simulink model "ball_and_plate_za_nn_2"  (R2018b)
settings: Solver=ode45  StartTime=0.0  StopTime=t_sim  RelTol=1e-3  EnableMultiTasking=on
values from neighbouring files (symbols this model uses):
  A_x = 0.05    [parametri.mat]    (also in proba_nn_simulink.m = 0.1; simulate_NOE_NARX_performance.mat = 0.1; simuliraj_kruznicu.m = radijus; test_nn_.m = 0.1)
  a_x = 0.388    [parametri.mat]    (also in simulate_NOE_NARX_performance.mat)
  A_y = 0.05    [parametri.mat]    (also in proba_nn_simulink.m = 0.1; simulate_NOE_NARX_performance.mat = 0.1; simuliraj_kruznicu.m = radijus; test_nn_.m = 0.1)
  a_y = 0.473    [parametri.mat]    (also in simulate_NOE_NARX_performance.mat)
  Ak_x = 0.1    [parametri.mat]    (also in simulate_NOE_NARX_performance.mat; simuliraj_kvadrat.m = stranica)
  Ak_y = 0.1    [parametri.mat]    (also in simulate_NOE_NARX_performance.mat; simuliraj_kvadrat.m = stranica)
  d = 2    [parametri.mat]    (also in simulate_NOE_NARX_performance.mat)
  Fc = 9.9675e-08    [parametri.mat]    (also in simulate_NOE_NARX_performance.mat)
  freq_x = 0.628318530718    [parametri.mat]    (also in simulate_NOE_NARX_performance.mat)
  freq_y = 0.628318530718    [parametri.mat]    (also in simulate_NOE_NARX_performance.mat)
  Fs = 1.9935e-07    [parametri.mat]    (also in simulate_NOE_NARX_performance.mat)
  g = 9.81    [parametri.mat]    (also in simulate_NOE_NARX_performance.mat)
  Jl = 7.48815837481e-05    [parametri.mat]    (also in simulate_NOE_NARX_performance.mat)
  konstanta = 0.1    [parametri.mat]    (also in simulate_NOE_NARX_performance.mat; simuliraj_kvadrat.m = 0.03)
  l = 0.1    [parametri.mat]    (also in simulate_NOE_NARX_performance.mat)
  ml = 0.0786597330257    [parametri.mat]    (also in simulate_NOE_NARX_performance.mat)
  odabir = 3    [proba_nn_simulink.m]    (also in simulate_NOE_NARX_performance.mat; simuliraj_kruznicu.m; simuliraj_kvadrat.m = 2; simuliraj_referenca.m = 1)
  period_x = 16    [parametri.mat]    (also in simulate_NOE_NARX_performance.mat)
  period_y = 16    [parametri.mat]    (also in simulate_NOE_NARX_performance.mat)
  phase_x = 1.57079632679    [parametri.mat]    (also in simulate_NOE_NARX_performance.mat)
  phase_y = 0    [parametri.mat]    (also in simulate_NOE_NARX_performance.mat)
  phasedelay_x = 0    [parametri.mat]    (also in simulate_NOE_NARX_performance.mat)
  phasedelay_y = 4    [parametri.mat]    (also in simulate_NOE_NARX_performance.mat)
  pw_x = 50    [parametri.mat]    (also in simulate_NOE_NARX_performance.mat)
  pw_y = 50    [parametri.mat]    (also in simulate_NOE_NARX_performance.mat)
  R = 0.0397    [parametri.mat]    (also in simulate_NOE_NARX_performance.mat)
  r = 0.02    [parametri.mat]    (also in simulate_NOE_NARX_performance.mat)
  t_step = 5    [parametri.mat]    (also in simulate_NOE_NARX_performance.mat)
  Td = 0.1    [parametri.mat]    (also in simulate_NOE_NARX_performance.mat)
  vs = 0.05    [parametri.mat]    (also in simulate_NOE_NARX_performance.mat)
  x0 = 0.15    [parametri.mat]    (also in proba_nn_simulink.m = a_x/2.0; simulate_NOE_NARX_performance.mat = 0.194; simuliraj_kruznicu.m = a_x/2.0; test_nn_.m = a_x/2.0)
  x0_loptica = 0.1    [proba_nn_simulink.m]    (also in simulate_NOE_NARX_performance.mat; simuliraj_kruznicu.m = x0_poc; simuliraj_kvadrat.m = x0_poc; simuliraj_referenca.m = x0_poc)
  x_step = 0.05    [parametri.mat]    (also in simulate_NOE_NARX_performance.mat; simuliraj_referenca.m = x_ref_value)
  y0 = 0.15    [parametri.mat]    (also in proba_nn_simulink.m = a_y/2.0; simulate_NOE_NARX_performance.mat = 0.2365; simuliraj_kruznicu.m = a_y/2.0; test_nn_.m = a_y/2.0)
  y0_loptica = 0.1    [proba_nn_simulink.m]    (also in simulate_NOE_NARX_performance.mat; simuliraj_kruznicu.m = y0_poc; simuliraj_kvadrat.m = y0_poc; simuliraj_referenca.m = y0_poc)
  y_step = 0.05    [parametri.mat]    (also in simulate_NOE_NARX_performance.mat; simuliraj_referenca.m = y_ref_value)
libraries: neural x118, simulink x6, fuzblock x2
(part 1 of 5)
settings Model: SimulationMode=accelerator  Creator=Damjan  LastModifiedBy=branko
settings DataIOCC: LimitDataPoints=on  SaveFormat=Array  SignalLoggingSaveFormat=ModelDataLogs
settings OptimizationCC: ExpressionDepthLimit=2147483647  LifeSpan=inf
settings DebuggingCC: UnderspecifiedInitializationDetection=Classic  MergeDetectMultiDrivingBlocksExec=none  FcnCallInpInsideContextMsg=warning  AllowSymbolicDim=off  StateNameClashWarn=warning  SFUnexpectedBacktrackingDiag=warning  SFNoUnconditionalDefaultTransitionDiag=warning  SFExecutionAtInitializationDiag=none
settings HardwareCC: ProdBitPerPointer=32  ProdBitPerSizeT=32  ProdBitPerPtrDiffT=32  ProdLargestAtomicFloat=None  ProdIntDivRoundTo=Undefined  ProdEndianess=Unspecified  ProdWordSize=32  ProdHWDeviceType=32-bit Generic
settings ModelReferenceCC: PropagateSignalLabelsOutOfModel=off
settings SFSimCC: SimUseLocalCustomCode=off
settings RTWCC: RTWUseLocalCustomCode=off
settings CodeAppCC: StateflowObjectComments=on
settings GRTTargetCC: TargetLangStandard=C89/C90 (ANSI)  GeneratePreprocessorConditionals=Disable all  CombineOutputUpdateFcns=off  GRTInterface=on
settings ConfigComp: CovMetricSettings=dw  CovHtmlReporting=on  CovSaveCumulativeToWorkspaceVar=on  CovSaveSingleToWorkspaceVar=on  CovExternalEMLEnable=off

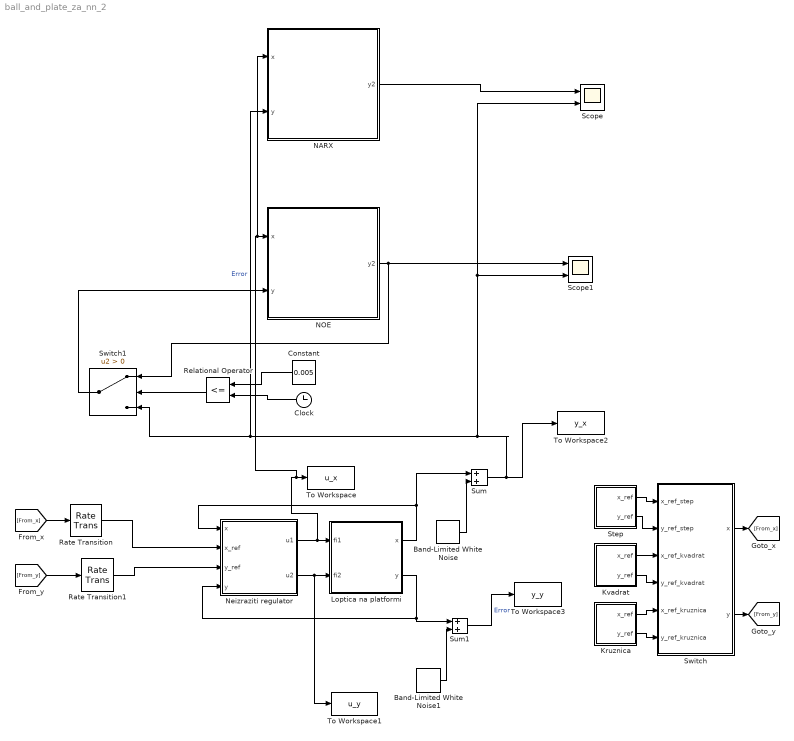
== system ball_and_plate_za_nn_2 ==
  Band-Limited White Noise : simulink/Sources/Band-Limited White Noise  Cov=[1e-9]  Ts=0.001  seed=[23341]
  Band-Limited White Noise1 : simulink/Sources/Band-Limited White Noise  Cov=[1e-9]  Ts=0.001  seed=[23341]
  Clock : Clock
  Constant : Constant  Value=0.005  OutDataTypeStr=double  SampleTime=-1
  Kruznica : Subsystem
  Kvadrat : Subsystem
  Loptica na platformi : Subsystem
  NARX : Subsystem  mask{pi_input_1_delayed_1=0, pi_input_1_delayed_2=0, pi_input_1_delayed_3=0, pi_input_1_delayed_4=0, pi_input_1_delayed_5=0, pi_input_2_delayed_1=0, pi_input_2_delayed_2=0, pi_input_2_delayed_3=0, pi_input_2_delayed_4=0, pi_input_2_delayed_5=0}
      mask prompts: pi_input_1_delayed_1 "Preprocessed initial input 1 state at timestep 0."; pi_input_1_delayed_2 "Preprocessed initial input 1 state at timestep -1."; pi_input_1_delayed_3 "Preprocessed initial input 1 state at timestep -2."; pi_input_1_delayed_4 "Preprocessed initial input 1 state at timestep -3."; pi_input_1_delayed_5 "Preprocessed initial input 1 state at timestep -4."; pi_input_2_delayed_1 "Preprocessed initial input 2 state at timestep 0."; pi_input_2_delayed_2 "Preprocessed initial input 2 state at timestep -1."; pi_input_2_delayed_3 "Preprocessed initial input 2 state at timestep -2."; pi_input_2_delayed_4 "Preprocessed initial input 2 state at timestep -3."; pi_input_2_delayed_5 "Preprocessed initial input 2 state at timestep -4."
      mask help: NARX Neural Network
      mask Display: e = 0.06;c1 = [120 150 230]/255;c2 = ([120 150 230]+0)/383;c3 = ([120 150 230]+128)/383;patch([0 1 1 0],[0 0 1 1],c1);patch([0 1 1 1-e 1-e 0+e],[0 0 1 1-e 0+e 0+e],c2);patch([0 0 1 1-e 0+e 0+e],[0 1 1 1-e 1-e 0+e],c3);plot([0 1 1 0 0],[0 0 1 1 0]);fprintf('NNET');port_label('input',1,' x');port_label('input',2,' y');port_label('output',1,'y2 ');
  NOE : Subsystem  mask{pi_input_1_delayed_1=0, pi_input_1_delayed_2=0, pi_input_1_delayed_3=0, pi_input_1_delayed_4=0, pi_input_1_delayed_5=0, pi_input_2_delayed_1=0, pi_input_2_delayed_2=0, pi_input_2_delayed_3=0, pi_input_2_delayed_4=0, pi_input_2_delayed_5=0}
      mask prompts: pi_input_1_delayed_1 "Preprocessed initial input 1 state at timestep 0."; pi_input_1_delayed_2 "Preprocessed initial input 1 state at timestep -1."; pi_input_1_delayed_3 "Preprocessed initial input 1 state at timestep -2."; pi_input_1_delayed_4 "Preprocessed initial input 1 state at timestep -3."; pi_input_1_delayed_5 "Preprocessed initial input 1 state at timestep -4."; pi_input_2_delayed_1 "Preprocessed initial input 2 state at timestep 0."; pi_input_2_delayed_2 "Preprocessed initial input 2 state at timestep -1."; pi_input_2_delayed_3 "Preprocessed initial input 2 state at timestep -2."; pi_input_2_delayed_4 "Preprocessed initial input 2 state at timestep -3."; pi_input_2_delayed_5 "Preprocessed initial input 2 state at timestep -4."
      mask help: NARX Neural Network
      mask Display: e = 0.06;c1 = [120 150 230]/255;c2 = ([120 150 230]+0)/383;c3 = ([120 150 230]+128)/383;patch([0 1 1 0],[0 0 1 1],c1);patch([0 1 1 1-e 1-e 0+e],[0 0 1 1-e 0+e 0+e],c2);patch([0 0 1 1-e 0+e 0+e],[0 1 1 1-e 1-e 0+e],c3);plot([0 1 1 0 0],[0 0 1 1 0]);fprintf('NNET');port_label('input',1,' x');port_label('input',2,' y');port_label('output',1,'y2 ');
  Neizraziti regulator : Subsystem
  Rate Transition : RateTransition  OutPortSampleTime=0.001
  Rate Transition1 : RateTransition  OutPortSampleTime=0.001
  Relational Operator : RelationalOperator  Operator=<=  OutDataTypeStr=boolean  RndMeth=Simplest
  Scope : Scope  NumInputPorts=2
  Scope1 : Scope  NumInputPorts=2
  Step : Subsystem
  Sum : Sum
  Sum1 : Sum
  Switch : Subsystem
  Switch1 : Switch  Criteria=u2 > Threshold
  To Workspace : ToWorkspace  VariableName=u_x  SaveFormat=Structure With Time  SampleTime=0.001
  To Workspace1 : ToWorkspace  VariableName=u_y  SaveFormat=Structure With Time  SampleTime=0.001
  To Workspace2 : ToWorkspace  VariableName=y_x  SaveFormat=Structure With Time  SampleTime=0.001
  To Workspace3 : ToWorkspace  VariableName=y_y  SaveFormat=Structure With Time  SampleTime=0.001
  wires:
  Loptica na platformi/1(x) -> Sum/1, Neizraziti regulator/1(x)
  Loptica na platformi/2(y) -> Sum1/1, Neizraziti regulator/4(y)
  Neizraziti regulator/1(u1) -> NARX/1(x), NOE/1(x), To Workspace/1, Loptica na platformi/1(fi1)
  Neizraziti regulator/2(u2) -> To Workspace1/1, Loptica na platformi/2(fi2)
  [From_x] -> Rate Transition/1
  [From_y] -> Rate Transition1/1
  Switch/1(x) -> [From_x]
  Switch/2(y) -> [From_y]
  Step/1(x_ref) -> Switch/1(x_ref_step)
  Step/2(y_ref) -> Switch/2(y_ref_step)
  Kvadrat/1(x_ref) -> Switch/3(x_ref_kvadrat)
  Kvadrat/2(y_ref) -> Switch/4(y_ref_kvadrat)
  Kruznica/1(x_ref) -> Switch/5(x_ref_kruznica)
  Kruznica/2(y_ref) -> Switch/6(y_ref_kruznica)
  Band-Limited White Noise/1 -> Sum/2
  Sum/1 -> Scope1/2, Scope/2, NARX/2(y), Switch1/3, To Workspace2/1  "Error"
  Band-Limited White Noise1/1 -> Sum1/2
  Sum1/1 -> To Workspace3/1  "Error"
  Constant/1 -> Relational Operator/1
  Clock/1 -> Relational Operator/2
  Relational Operator/1 -> Switch1/2
  NOE/1(y2) -> Scope1/1, Switch1/1
  Switch1/1 -> NOE/2(y)
  Rate Transition/1 -> Neizraziti regulator/2(x_ref)
  Rate Transition1/1 -> Neizraziti regulator/3(y_ref)
  NARX/1(y2) -> Scope/1

== system ball_and_plate_za_nn_2/Kruznica ==
  Sinus x : Sin  Amplitude=A_x  Bias=x0  Frequency=freq_x  Phase=phase_x  SampleTime=0
  Sinus y : Sin  Amplitude=A_y  Bias=y0  Frequency=freq_y  Phase=phase_y  SampleTime=0
  x_ref : Outport
  y_ref : Outport  Port=2
  wires:
  Sinus x/1 -> x_ref/1
  Sinus y/1 -> y_ref/1

== system ball_and_plate_za_nn_2/Kvadrat ==
  Pulse Generator_x : DiscretePulseGenerator  PulseType=Time based  Amplitude=Ak_x  Period=period_x  PulseWidth=pw_x  PhaseDelay=phasedelay_x
  Pulse Generator_y : DiscretePulseGenerator  PulseType=Time based  Amplitude=Ak_y  Period=period_y  PulseWidth=pw_y  PhaseDelay=phasedelay_y
  Sum : Sum  Inputs=|++
  Sum1 : Sum  Inputs=|++
  const : Constant  Value=konstanta
  x_ref : Outport
  y_ref : Outport  Port=2
  wires:
  Sum/1 -> x_ref/1
  Sum1/1 -> y_ref/1
  Pulse Generator_x/1 -> Sum/1
  Pulse Generator_y/1 -> Sum1/1
  const/1 -> Sum1/2, Sum/2

== system ball_and_plate_za_nn_2/Loptica na platformi ==
  fi1 : Inport
  fi2 : Inport  Port=2
  Loptica : Subsystem
  Platforma : Subsystem
  x : Outport
  y : Outport  Port=2
  wires:
  Loptica/1(x) -> x/1
  fi1/1 -> Platforma/1(fi1)
  fi2/1 -> Platforma/2(fi2)
  Loptica/2(y) -> y/1
  Platforma/2(alfa) -> Loptica/2(alfa)
  Platforma/1(beta) -> Loptica/1(beta)

== system ball_and_plate_za_nn_2/NARX ==
  x : Inport  PortDimensions=1  SampleTime=0.001
      mask Display: e = 0.06;c1 = [120 230 180]/255;c2 = ([120 230 180]+0)/(256+128);c3 = ([120 230 180]+128)/(256+128);patch([0 1 1 0],[0 0 1 1],c1);patch([0 1 1 1-e 1-e 0+e],[0 0 1 1-e 0+e 0+e],c2);patch([0 0 1 1-e 0+e 0+e],[0 1 1 1-e 1-e 0+e],c3);plot([0 1 1 0 0],[0 0 1 1 0]);
  y : Inport  Port=2  PortDimensions=1  SampleTime=0.001
      mask Display: e = 0.06;c1 = [120 230 180]/255;c2 = ([120 230 180]+0)/(256+128);c3 = ([120 230 180]+128)/(256+128);patch([0 1 1 0],[0 0 1 1],c1);patch([0 1 1 1-e 1-e 0+e],[0 0 1 1-e 0+e 0+e],c2);patch([0 0 1 1-e 0+e 0+e],[0 1 1 1-e 1-e 0+e],c3);plot([0 1 1 0 0],[0 0 1 1 0]);
  Layer 1 : Subsystem
      mask Display: e = 0.06;c1 = [120 150 230]/255;c2 = ([120 150 230]+0)/383;c3 = ([120 150 230]+128)/383;patch([0 1 1 0],[0 0 1 1],c1);patch([0 1 1 1-e 1-e 0+e],[0 0 1 1-e 0+e 0+e],c2);patch([0 0 1 1-e 0+e 0+e],[0 1 1 1-e 1-e 0+e],c3);plot([0 1 1 0 0],[0 0 1 1 0]);
  Layer 2 : Subsystem
      mask Display: e = 0.06;c1 = [120 150 230]/255;c2 = ([120 150 230]+0)/383;c3 = ([120 150 230]+128)/383;patch([0 1 1 0],[0 0 1 1],c1);patch([0 1 1 1-e 1-e 0+e],[0 0 1 1-e 0+e 0+e],c2);patch([0 0 1 1-e 0+e 0+e],[0 1 1 1-e 1-e 0+e],c3);plot([0 1 1 0 0],[0 0 1 1 0]);
  Layer 3 : Subsystem
      mask Display: e = 0.06;c1 = [120 150 230]/255;c2 = ([120 150 230]+0)/383;c3 = ([120 150 230]+128)/383;patch([0 1 1 0],[0 0 1 1],c1);patch([0 1 1 1-e 1-e 0+e],[0 0 1 1-e 0+e 0+e],c2);patch([0 0 1 1-e 0+e 0+e],[0 1 1 1-e 1-e 0+e],c3);plot([0 1 1 0 0],[0 0 1 1 0]);
  Layer 4 : Subsystem
      mask Display: e = 0.06;c1 = [120 150 230]/255;c2 = ([120 150 230]+0)/383;c3 = ([120 150 230]+128)/383;patch([0 1 1 0],[0 0 1 1],c1);patch([0 1 1 1-e 1-e 0+e],[0 0 1 1-e 0+e 0+e],c2);patch([0 0 1 1-e 0+e 0+e],[0 1 1 1-e 1-e 0+e],c3);plot([0 1 1 0 0],[0 0 1 1 0]);
  Layer 5 : Subsystem
      mask Display: e = 0.06;c1 = [120 150 230]/255;c2 = ([120 150 230]+0)/383;c3 = ([120 150 230]+128)/383;patch([0 1 1 0],[0 0 1 1],c1);patch([0 1 1 1-e 1-e 0+e],[0 0 1 1-e 0+e 0+e],c2);patch([0 0 1 1-e 0+e 0+e],[0 1 1 1-e 1-e 0+e],c3);plot([0 1 1 0 0],[0 0 1 1 0]);
  Process Input 1 : Subsystem
      mask Display: e = 0.06;c1 = [120 150 230]/255;c2 = ([120 150 230]+0)/383;c3 = ([120 150 230]+128)/383;patch([0 1 1 0],[0 0 1 1],c1);patch([0 1 1 1-e 1-e 0+e],[0 0 1 1-e 0+e 0+e],c2);patch([0 0 1 1-e 0+e 0+e],[0 1 1 1-e 1-e 0+e],c3);plot([0 1 1 0 0],[0 0 1 1 0]);
  Process Input 2 : Subsystem
      mask Display: e = 0.06;c1 = [120 150 230]/255;c2 = ([120 150 230]+0)/383;c3 = ([120 150 230]+128)/383;patch([0 1 1 0],[0 0 1 1],c1);patch([0 1 1 1-e 1-e 0+e],[0 0 1 1-e 0+e 0+e],c2);patch([0 0 1 1-e 0+e 0+e],[0 1 1 1-e 1-e 0+e],c3);plot([0 1 1 0 0],[0 0 1 1 0]);
  Process Output 1 : Subsystem
      mask Display: e = 0.06;c1 = [120 150 230]/255;c2 = ([120 150 230]+0)/383;c3 = ([120 150 230]+128)/383;patch([0 1 1 0],[0 0 1 1],c1);patch([0 1 1 1-e 1-e 0+e],[0 0 1 1-e 0+e 0+e],c2);patch([0 0 1 1-e 0+e 0+e],[0 1 1 1-e 1-e 0+e],c3);plot([0 1 1 0 0],[0 0 1 1 0]);
  y2 : Outport  InitialOutput=0
      mask Display: e = 0.06;c1 = [120 230 180]/255;c2 = ([120 230 180]+0)/(256+128);c3 = ([120 230 180]+128)/(256+128);patch([0 1 1 0],[0 0 1 1],c1);patch([0 1 1 1-e 1-e 0+e],[0 0 1 1-e 0+e 0+e],c2);patch([0 0 1 1-e 0+e 0+e],[0 1 1 1-e 1-e 0+e],c3);plot([0 1 1 0 0],[0 0 1 1 0]);
  wires:
  x/1 -> Process Input 1/1(x)
  y/1 -> Process Input 2/1(x)
  Process Output 1/1(y) -> y2/1
  Process Input 1/1(p) -> Layer 1/1("p{1}")
  Process Input 2/1(p) -> Layer 1/2("p{2}")
  Layer 1/1("a{1}") -> [feedback1]
  [feedback1] -> Layer 2/1("a{1} ")
  Layer 2/1("a{2}") -> [feedback2]
  [feedback2] -> Layer 3/1("a{2} ")
  Layer 3/1("a{3}") -> [feedback3]
  [feedback3] -> Layer 4/1("a{3} ")
  Layer 4/1("a{4}") -> [feedback4]
  [feedback4] -> Layer 5/1("a{4} ")
  Layer 5/1("a{5}") -> Process Output 1/1(a)

== system ball_and_plate_za_nn_2/NOE ==
  x : Inport  PortDimensions=1  SampleTime=0.001
      mask Display: e = 0.06;c1 = [120 230 180]/255;c2 = ([120 230 180]+0)/(256+128);c3 = ([120 230 180]+128)/(256+128);patch([0 1 1 0],[0 0 1 1],c1);patch([0 1 1 1-e 1-e 0+e],[0 0 1 1-e 0+e 0+e],c2);patch([0 0 1 1-e 0+e 0+e],[0 1 1 1-e 1-e 0+e],c3);plot([0 1 1 0 0],[0 0 1 1 0]);
  y : Inport  Port=2  PortDimensions=1  SampleTime=0.001
      mask Display: e = 0.06;c1 = [120 230 180]/255;c2 = ([120 230 180]+0)/(256+128);c3 = ([120 230 180]+128)/(256+128);patch([0 1 1 0],[0 0 1 1],c1);patch([0 1 1 1-e 1-e 0+e],[0 0 1 1-e 0+e 0+e],c2);patch([0 0 1 1-e 0+e 0+e],[0 1 1 1-e 1-e 0+e],c3);plot([0 1 1 0 0],[0 0 1 1 0]);
  Layer 1 : Subsystem
      mask Display: e = 0.06;c1 = [120 150 230]/255;c2 = ([120 150 230]+0)/383;c3 = ([120 150 230]+128)/383;patch([0 1 1 0],[0 0 1 1],c1);patch([0 1 1 1-e 1-e 0+e],[0 0 1 1-e 0+e 0+e],c2);patch([0 0 1 1-e 0+e 0+e],[0 1 1 1-e 1-e 0+e],c3);plot([0 1 1 0 0],[0 0 1 1 0]);
  Layer 2 : Subsystem
      mask Display: e = 0.06;c1 = [120 150 230]/255;c2 = ([120 150 230]+0)/383;c3 = ([120 150 230]+128)/383;patch([0 1 1 0],[0 0 1 1],c1);patch([0 1 1 1-e 1-e 0+e],[0 0 1 1-e 0+e 0+e],c2);patch([0 0 1 1-e 0+e 0+e],[0 1 1 1-e 1-e 0+e],c3);plot([0 1 1 0 0],[0 0 1 1 0]);
  Layer 3 : Subsystem
      mask Display: e = 0.06;c1 = [120 150 230]/255;c2 = ([120 150 230]+0)/383;c3 = ([120 150 230]+128)/383;patch([0 1 1 0],[0 0 1 1],c1);patch([0 1 1 1-e 1-e 0+e],[0 0 1 1-e 0+e 0+e],c2);patch([0 0 1 1-e 0+e 0+e],[0 1 1 1-e 1-e 0+e],c3);plot([0 1 1 0 0],[0 0 1 1 0]);
  Layer 4 : Subsystem
      mask Display: e = 0.06;c1 = [120 150 230]/255;c2 = ([120 150 230]+0)/383;c3 = ([120 150 230]+128)/383;patch([0 1 1 0],[0 0 1 1],c1);patch([0 1 1 1-e 1-e 0+e],[0 0 1 1-e 0+e 0+e],c2);patch([0 0 1 1-e 0+e 0+e],[0 1 1 1-e 1-e 0+e],c3);plot([0 1 1 0 0],[0 0 1 1 0]);
  Layer 5 : Subsystem
      mask Display: e = 0.06;c1 = [120 150 230]/255;c2 = ([120 150 230]+0)/383;c3 = ([120 150 230]+128)/383;patch([0 1 1 0],[0 0 1 1],c1);patch([0 1 1 1-e 1-e 0+e],[0 0 1 1-e 0+e 0+e],c2);patch([0 0 1 1-e 0+e 0+e],[0 1 1 1-e 1-e 0+e],c3);plot([0 1 1 0 0],[0 0 1 1 0]);
  Process Input 1 : Subsystem
      mask Display: e = 0.06;c1 = [120 150 230]/255;c2 = ([120 150 230]+0)/383;c3 = ([120 150 230]+128)/383;patch([0 1 1 0],[0 0 1 1],c1);patch([0 1 1 1-e 1-e 0+e],[0 0 1 1-e 0+e 0+e],c2);patch([0 0 1 1-e 0+e 0+e],[0 1 1 1-e 1-e 0+e],c3);plot([0 1 1 0 0],[0 0 1 1 0]);
  Process Input 2 : Subsystem
      mask Display: e = 0.06;c1 = [120 150 230]/255;c2 = ([120 150 230]+0)/383;c3 = ([120 150 230]+128)/383;patch([0 1 1 0],[0 0 1 1],c1);patch([0 1 1 1-e 1-e 0+e],[0 0 1 1-e 0+e 0+e],c2);patch([0 0 1 1-e 0+e 0+e],[0 1 1 1-e 1-e 0+e],c3);plot([0 1 1 0 0],[0 0 1 1 0]);
  Process Output 1 : Subsystem
      mask Display: e = 0.06;c1 = [120 150 230]/255;c2 = ([120 150 230]+0)/383;c3 = ([120 150 230]+128)/383;patch([0 1 1 0],[0 0 1 1],c1);patch([0 1 1 1-e 1-e 0+e],[0 0 1 1-e 0+e 0+e],c2);patch([0 0 1 1-e 0+e 0+e],[0 1 1 1-e 1-e 0+e],c3);plot([0 1 1 0 0],[0 0 1 1 0]);
  y2 : Outport  InitialOutput=0
      mask Display: e = 0.06;c1 = [120 230 180]/255;c2 = ([120 230 180]+0)/(256+128);c3 = ([120 230 180]+128)/(256+128);patch([0 1 1 0],[0 0 1 1],c1);patch([0 1 1 1-e 1-e 0+e],[0 0 1 1-e 0+e 0+e],c2);patch([0 0 1 1-e 0+e 0+e],[0 1 1 1-e 1-e 0+e],c3);plot([0 1 1 0 0],[0 0 1 1 0]);
  wires:
  x/1 -> Process Input 1/1(x)
  y/1 -> Process Input 2/1(x)
  Process Output 1/1(y) -> y2/1
  Process Input 1/1(p) -> Layer 1/1("p{1}")
  Process Input 2/1(p) -> Layer 1/2("p{2}")
  Layer 1/1("a{1}") -> [feedback1]
  [feedback1] -> Layer 2/1("a{1} ")
  Layer 2/1("a{2}") -> [feedback2]
  [feedback2] -> Layer 3/1("a{2} ")
  Layer 3/1("a{3}") -> [feedback3]
  [feedback3] -> Layer 4/1("a{3} ")
  Layer 4/1("a{4}") -> [feedback4]
  [feedback4] -> Layer 5/1("a{4} ")
  Layer 5/1("a{5}") -> Process Output 1/1(a)

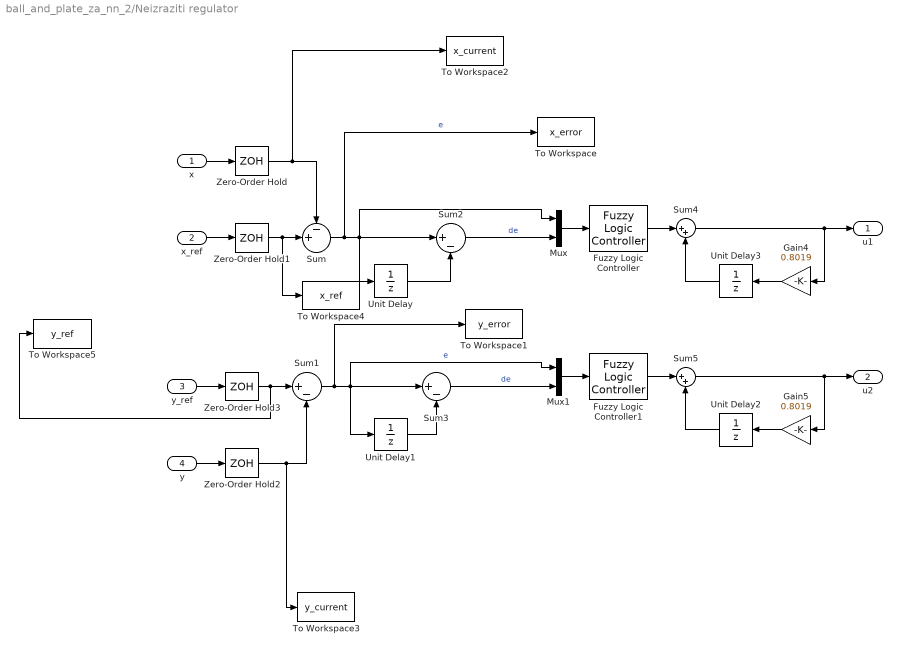
== system ball_and_plate_za_nn_2/Neizraziti regulator ==
  x : Inport
  x_ref : Inport  Port=2
  y_ref : Inport  Port=3
  y : Inport  Port=4
  Fuzzy Logic Controller : fuzblock/Fuzzy Logic  Controller  FIS=fuzzy_FIS  OutputSampleNumber=101  DataType=double  FuzzifiedInputs=off  RuleFiringStrengths=off  RuleOutputs=off  AggregatedOutputs=off  SimulateUsing=Interpreted execution  OutOfRangeInputValueMessage=warning  NoRuleFiredMessage=warning  EmptyOutputFuzzySetMessage=warning
  Fuzzy Logic Controller1 : fuzblock/Fuzzy Logic  Controller  FIS=fuzzy_FIS  OutputSampleNumber=101  DataType=double  FuzzifiedInputs=off  RuleFiringStrengths=off  RuleOutputs=off  AggregatedOutputs=off  SimulateUsing=Interpreted execution  OutOfRangeInputValueMessage=warning  NoRuleFiredMessage=warning  EmptyOutputFuzzySetMessage=warning
  Gain4 : Gain  Gain=0.8019
  Gain5 : Gain  Gain=0.8019
  Mux : Mux  Inputs=2
  Mux1 : Mux  Inputs=2
  Sum : Sum  Inputs=-+|  RndMeth=Nearest
  Sum1 : Sum  Inputs=|+-  RndMeth=Nearest
  Sum2 : Sum  Inputs=|+-
  Sum3 : Sum  Inputs=|+-
  Sum4 : Sum  Inputs=|++
  Sum5 : Sum  Inputs=|++
  To Workspace : ToWorkspace  VariableName=x_error  SaveFormat=Structure With Time  SampleTime=0.001
  To Workspace1 : ToWorkspace  VariableName=y_error  SaveFormat=Structure With Time  SampleTime=0.001
  To Workspace2 : ToWorkspace  VariableName=x_current  SaveFormat=Structure With Time  SampleTime=0.001
  To Workspace3 : ToWorkspace  VariableName=y_current  SaveFormat=Structure With Time  SampleTime=0.001
  To Workspace4 : ToWorkspace  VariableName=x_ref  SaveFormat=Structure With Time  SampleTime=0.001
  To Workspace5 : ToWorkspace  VariableName=y_ref  SaveFormat=Structure With Time  SampleTime=0.001
  Unit Delay : UnitDelay  SampleTime=-1
  Unit Delay1 : UnitDelay  SampleTime=-1
  Unit Delay2 : UnitDelay  SampleTime=Td
  Unit Delay3 : UnitDelay  SampleTime=Td
  Zero-Order Hold{,1..3} (4 alike) : ZeroOrderHold  SampleTime=Td
  u1 : Outport
  u2 : Outport  Port=2
  wires:
  x/1 -> Zero-Order Hold/1
  x_ref/1 -> Zero-Order Hold1/1
  y_ref/1 -> Zero-Order Hold3/1
  y/1 -> Zero-Order Hold2/1
  Zero-Order Hold/1 -> To Workspace2/1, Sum/1
  Zero-Order Hold1/1 -> To Workspace4/1, Sum/2
  Zero-Order Hold3/1 -> To Workspace5/1, Sum1/1
  Zero-Order Hold2/1 -> To Workspace3/1, Sum1/2
  Sum/1 -> To Workspace/1, Sum2/1, Unit Delay/1, Mux/1  "e"
  Sum2/1 -> Mux/2  "de"
  Sum3/1 -> Mux1/2  "de"
  Sum4/1 -> u1/1, Gain4/1
  Sum5/1 -> u2/1, Gain5/1
  Unit Delay3/1 -> Sum4/2
  Unit Delay2/1 -> Sum5/2
  Gain4/1 -> Unit Delay3/1
  Gain5/1 -> Unit Delay2/1
  Fuzzy Logic Controller/1 -> Sum4/1
  Fuzzy Logic Controller1/1 -> Sum5/1
  Unit Delay/1 -> Sum2/2
  Mux/1 -> Fuzzy Logic Controller/1
  Unit Delay1/1 -> Sum3/2
  Mux1/1 -> Fuzzy Logic Controller1/1
  Sum1/1 -> To Workspace1/1, Sum3/1, Unit Delay1/1, Mux1/1  "e"

== system ball_and_plate_za_nn_2/Step ==
  xRef Step : Step  Time=t_step  Before=x0_loptica  After=x_step  SampleTime=0
  yRef Step : Step  Time=t_step  Before=y0_loptica  After=y_step  SampleTime=0
  x_ref : Outport
  y_ref : Outport  Port=2
  wires:
  xRef Step/1 -> x_ref/1
  yRef Step/1 -> y_ref/1

== system ball_and_plate_za_nn_2/Switch ==
  x_ref_step : Inport
  y_ref_step : Inport  Port=2
  x_ref_kvadrat : Inport  Port=3
  y_ref_kvadrat : Inport  Port=4
  x_ref_kruznica : Inport  Port=5
  y_ref_kruznica : Inport  Port=6
  Const_x : Constant  Value=odabir
  Const_y : Constant  Value=odabir
  Switch_x : MultiPortSwitch  DiagnosticForDefault=None
  Switch_y : MultiPortSwitch  DiagnosticForDefault=None
  x : Outport
  y : Outport  Port=2
  wires:
  Switch_x/1 -> x/1
  Switch_y/1 -> y/1
  x_ref_step/1 -> Switch_x/2
  x_ref_kvadrat/1 -> Switch_x/3
  x_ref_kruznica/1 -> Switch_x/4
  y_ref_kruznica/1 -> Switch_y/4
  y_ref_kvadrat/1 -> Switch_y/3
  y_ref_step/1 -> Switch_y/2
  Const_x/1 -> Switch_x/1
  Const_y/1 -> Switch_y/1

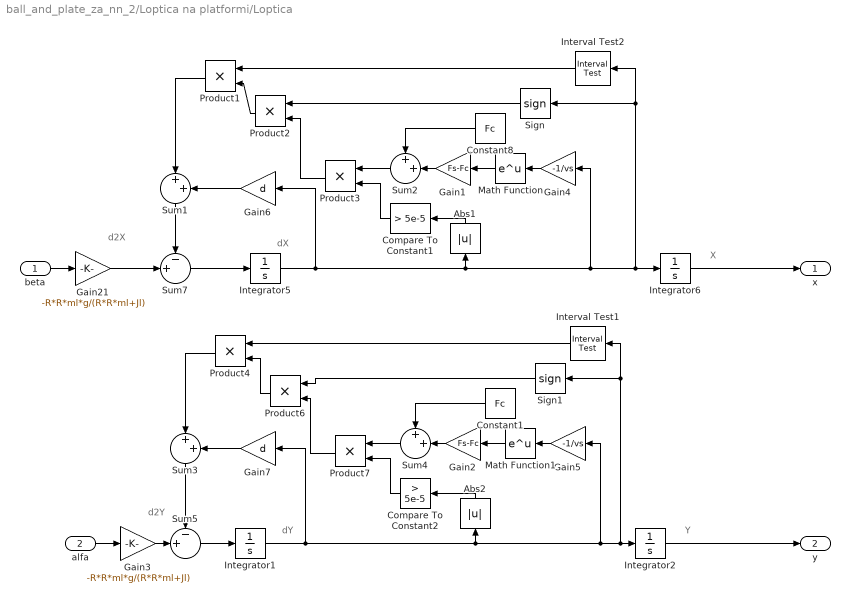
== system ball_and_plate_za_nn_2/Loptica na platformi/Loptica ==
  note: d2X
  note: dX
  note: X
  note: d2Y
  note: dY
  note: Y
  beta : Inport
  alfa : Inport  Port=2
  Abs1 : Abs
  Abs2 : Abs
  Compare To Constant1 : simulink/Logic and Bit Operations/Compare To Constant  relop=>  const=5e-5  OutDataTypeStr=boolean  ZeroCross=off
  Compare To Constant2 : simulink/Logic and Bit Operations/Compare To Constant  relop=>  const=5e-5  OutDataTypeStr=boolean  ZeroCross=off
  Constant1 : Constant  Value=Fc  SampleTime=0
  Constant8 : Constant  Value=Fc  SampleTime=0
  Gain1 : Gain  Gain=Fs-Fc  OutDataTypeStr=Inherit: Same as input  ParamDataTypeStr=Inherit: Same as input
  Gain2 : Gain  Gain=Fs-Fc  OutDataTypeStr=Inherit: Same as input  ParamDataTypeStr=Inherit: Same as input
  Gain21 : Gain  Gain=-R*R*ml*g/(R*R*ml+Jl)
  Gain3 : Gain  Gain=-R*R*ml*g/(R*R*ml+Jl)
  Gain4 : Gain  Gain=-1/vs  OutDataTypeStr=Inherit: Same as input  ParamDataTypeStr=Inherit: Same as input
  Gain5 : Gain  Gain=-1/vs  OutDataTypeStr=Inherit: Same as input  ParamDataTypeStr=Inherit: Same as input
  Gain6 : Gain  Gain=d  OutDataTypeStr=Inherit: Same as input  ParamDataTypeStr=Inherit: Same as input
  Gain7 : Gain  Gain=d  OutDataTypeStr=Inherit: Same as input  ParamDataTypeStr=Inherit: Same as input
  Integrator1 : Integrator
  Integrator2 : Integrator  InitialCondition=y0_loptica
  Integrator5 : Integrator
  Integrator6 : Integrator  InitialCondition=x0_loptica
  Interval Test1 : simulink/Logic and Bit Operations/Interval Test  IntervalClosedRight=on  uplimit=5e-5  IntervalClosedLeft=on  lowlimit=-5e-5  OutDataTypeStr=boolean
  Interval Test2 : simulink/Logic and Bit Operations/Interval Test  IntervalClosedRight=on  uplimit=5e-5  IntervalClosedLeft=on  lowlimit=-5e-5  OutDataTypeStr=boolean
  Math Function : Math  SaturateOnIntegerOverflow=on
  Math Function1 : Math  SaturateOnIntegerOverflow=on
  Product{1..4,6..7} (6 alike) : Product  RndMeth=Zero
  Sign : Signum
  Sign1 : Signum
  Sum1 : Sum  Inputs=|++
  Sum2 : Sum  Inputs=++|
  Sum3 : Sum  Inputs=|++
  Sum4 : Sum  Inputs=++|
  Sum5 : Sum  Inputs=-+|
  Sum7 : Sum  Inputs=-+|
  x : Outport
  y : Outport  Port=2
  wires:
  beta/1 -> Gain21/1
  Integrator5/1 -> Gain6/1, Integrator6/1, Interval Test2/1, Sign/1, Gain4/1, Abs1/1
  Sum7/1 -> Integrator5/1
  Gain4/1 -> Math Function/1
  Math Function/1 -> Gain1/1
  Gain1/1 -> Sum2/2
  Constant8/1 -> Sum2/1
  Sign/1 -> Product2/1
  Abs1/1 -> Compare To Constant1/1
  Sum2/1 -> Product3/1
  Compare To Constant1/1 -> Product3/2
  Product3/1 -> Product2/2
  Integrator1/1 -> Integrator2/1, Sign1/1, Interval Test1/1, Gain5/1, Abs2/1, Gain7/1
  Gain3/1 -> Sum5/2
  Sum5/1 -> Integrator1/1
  Gain5/1 -> Math Function1/1
  Math Function1/1 -> Gain2/1
  Gain2/1 -> Sum4/2
  Constant1/1 -> Sum4/1
  Sign1/1 -> Product6/1
  Abs2/1 -> Compare To Constant2/1
  Sum4/1 -> Product7/1
  Compare To Constant2/1 -> Product7/2
  Product7/1 -> Product6/2
  alfa/1 -> Gain3/1
  Integrator6/1 -> x/1
  Integrator2/1 -> y/1
  Interval Test2/1 -> Product1/1
  Product2/1 -> Product1/2
  Gain21/1 -> Sum7/2
  Product6/1 -> Product4/2
  Interval Test1/1 -> Product4/1
  Gain6/1 -> Sum1/2
  Sum1/1 -> Sum7/1
  Gain7/1 -> Sum3/2
  Sum3/1 -> Sum5/1
  Product1/1 -> Sum1/1
  Product4/1 -> Sum3/1

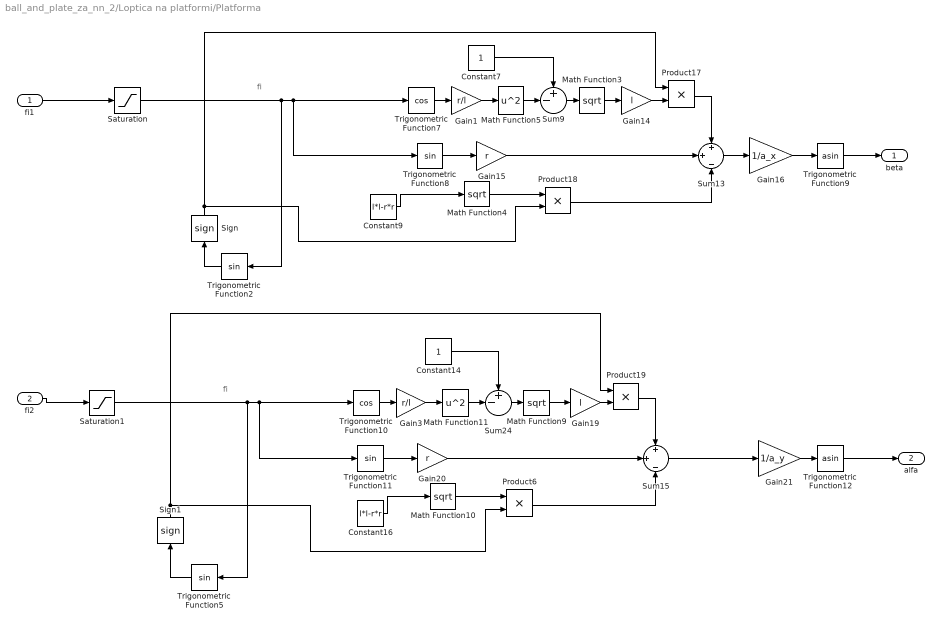
== system ball_and_plate_za_nn_2/Loptica na platformi/Platforma ==
  note: fi
  note: fi
  fi1 : Inport
  fi2 : Inport  Port=2
  Constant14 : Constant  SampleTime=0
  Constant16 : Constant  Value=l*l-r*r  SampleTime=0
  Constant7 : Constant  SampleTime=0
  Constant9 : Constant  Value=l*l-r*r  SampleTime=0
  Gain1 : Gain  Gain=r/l
  Gain14 : Gain  Gain=l
  Gain15 : Gain  Gain=r
  Gain16 : Gain  Gain=1/a_x
  Gain19 : Gain  Gain=l
  Gain20 : Gain  Gain=r
  Gain21 : Gain  Gain=1/a_y
  Gain3 : Gain  Gain=r/l
  Math Function{3..4,9..10} (4 alike) : Math  Operator=sqrt  SaturateOnIntegerOverflow=on
  Math Function11 : Math  Operator=square  SaturateOnIntegerOverflow=on
  Math Function5 : Math  Operator=square  SaturateOnIntegerOverflow=on
  Product{6,17..19} (4 alike) : Product  RndMeth=Zero
  Saturation : Saturate  UpperLimit=pi/2  LowerLimit=-pi/2
  Saturation1 : Saturate  UpperLimit=pi/2  LowerLimit=-pi/2
  Sign : Signum  ZeroCross=off
  Sign1 : Signum  ZeroCross=off
  Sum13 : Sum  Inputs=+|+|-  InputSameDT=on
  Sum15 : Sum  Inputs=+|+|-  InputSameDT=on
  Sum24 : Sum  Inputs=+-|
  Sum9 : Sum  Inputs=+-|
  Trigonometric Function10 : Trigonometry  Operator=cos
  Trigonometric Function{2,5,8,11} (4 alike) : Trigonometry
  Trigonometric Function12 : Trigonometry  Operator=asin
  Trigonometric Function7 : Trigonometry  Operator=cos
  Trigonometric Function9 : Trigonometry  Operator=asin
  beta : Outport
  alfa : Outport  Port=2
  wires:
  fi1/1 -> Saturation/1
  Trigonometric Function2/1 -> Sign/1
  Sign/1 -> Product18/2, Product17/1
  Trigonometric Function7/1 -> Gain1/1
  Constant7/1 -> Sum9/1
  Gain1/1 -> Math Function5/1
  Sum9/1 -> Math Function3/1
  Math Function3/1 -> Gain14/1
  Trigonometric Function8/1 -> Gain15/1
  Gain15/1 -> Sum13/2
  Constant9/1 -> Math Function4/1
  Gain16/1 -> Trigonometric Function9/1
  Math Function5/1 -> Sum9/2
  Sum13/1 -> Gain16/1
  Trigonometric Function5/1 -> Sign1/1
  Sign1/1 -> Product6/2, Product19/1
  Trigonometric Function10/1 -> Gain3/1
  Constant14/1 -> Sum24/1
  Gain3/1 -> Math Function11/1
  Sum24/1 -> Math Function9/1
  Math Function9/1 -> Gain19/1
  Trigonometric Function11/1 -> Gain20/1
  Gain20/1 -> Sum15/2
  Constant16/1 -> Math Function10/1
  Math Function11/1 -> Sum24/2
  Gain21/1 -> Trigonometric Function12/1
  Product17/1 -> Sum13/1
  Gain14/1 -> Product17/2
  Product18/1 -> Sum13/3
  Math Function4/1 -> Product18/1
  Product19/1 -> Sum15/1
  Gain19/1 -> Product19/2
  Product6/1 -> Sum15/3
  Math Function10/1 -> Product6/1
  Sum15/1 -> Gain21/1
  fi2/1 -> Saturation1/1
  Trigonometric Function9/1 -> beta/1
  Trigonometric Function12/1 -> alfa/1
  Saturation/1 -> Trigonometric Function7/1, Trigonometric Function8/1, Trigonometric Function2/1
  Saturation1/1 -> Trigonometric Function11/1, Trigonometric Function10/1, Trigonometric Function5/1

== system ball_and_plate_za_nn_2/NARX/Layer 1 ==
  "p{1}" : Inport  PortDimensions=1  SampleTime=0.001
      mask Display: e = 0.06;c1 = [120 230 180]/255;c2 = ([120 230 180]+0)/(256+128);c3 = ([120 230 180]+128)/(256+128);patch([0 1 1 0],[0 0 1 1],c1);patch([0 1 1 1-e 1-e 0+e],[0 0 1 1-e 0+e 0+e],c2);patch([0 0 1 1-e 0+e 0+e],[0 1 1 1-e 1-e 0+e],c3);plot([0 1 1 0 0],[0 0 1 1 0]);
  "p{2}" : Inport  Port=2  PortDimensions=1  SampleTime=0.001
      mask Display: e = 0.06;c1 = [120 230 180]/255;c2 = ([120 230 180]+0)/(256+128);c3 = ([120 230 180]+128)/(256+128);patch([0 1 1 0],[0 0 1 1],c1);patch([0 1 1 1-e 1-e 0+e],[0 0 1 1-e 0+e 0+e],c2);patch([0 0 1 1-e 0+e 0+e],[0 1 1 1-e 1-e 0+e],c3);plot([0 1 1 0 0],[0 0 1 1 0]);
  Delays 1 : Subsystem
      mask Display: e = 0.06;c1 = [120 150 230]/255;c2 = ([120 150 230]+0)/383;c3 = ([120 150 230]+128)/383;patch([0 1 1 0],[0 0 1 1],c1);patch([0 1 1 1-e 1-e 0+e],[0 0 1 1-e 0+e 0+e],c2);patch([0 0 1 1-e 0+e 0+e],[0 1 1 1-e 1-e 0+e],c3);plot([0 1 1 0 0],[0 0 1 1 0]);disp('1-5');
  Delays 2 : Subsystem
      mask Display: e = 0.06;c1 = [120 150 230]/255;c2 = ([120 150 230]+0)/383;c3 = ([120 150 230]+128)/383;patch([0 1 1 0],[0 0 1 1],c1);patch([0 1 1 1-e 1-e 0+e],[0 0 1 1-e 0+e 0+e],c2);patch([0 0 1 1-e 0+e 0+e],[0 1 1 1-e 1-e 0+e],c3);plot([0 1 1 0 0],[0 0 1 1 0]);disp('1-5');
  "IW{1,1}" : Subsystem
      mask Display: e = 0.06;c1 = [120 150 230]/255;c2 = ([120 150 230]+0)/383;c3 = ([120 150 230]+128)/383;patch([0 1 1 0],[0 0 1 1],c1);patch([0 1 1 1-e 1-e 0+e],[0 0 1 1-e 0+e 0+e],c2);patch([0 0 1 1-e 0+e 0+e],[0 1 1 1-e 1-e 0+e],c3);plot([0 1 1 0 0],[0 0 1 1 0]);disp('W');
  "IW{1,2}" : Subsystem
      mask Display: e = 0.06;c1 = [120 150 230]/255;c2 = ([120 150 230]+0)/383;c3 = ([120 150 230]+128)/383;patch([0 1 1 0],[0 0 1 1],c1);patch([0 1 1 1-e 1-e 0+e],[0 0 1 1-e 0+e 0+e],c2);patch([0 0 1 1-e 0+e 0+e],[0 1 1 1-e 1-e 0+e],c3);plot([0 1 1 0 0],[0 0 1 1 0]);disp('W');
  "b{1}" : Constant  Value=[1.8420085065380951139246690217987634241580963134765625;-1.6317189923451882460625483872718177735805511474609375;-0.78080933606115199285824246544507332146167755126953125;-0.90957261639388164997654939725180156528949737548828125;0.0509968115250476750066610520661924965679645538330078125;0.2969327933752257120403328372049145400524139404296875;0.76669410321683806319725817957078106701374053955078125;0.95673621890134319389886741191730834543704986572265625;1.540252046758102455470407221582718193531036376953125;-1.8537521132238807819447856672923080623149871826171875]
      mask Display: e = 0.06;c1 = [120 150 230]/255;c2 = ([120 150 230]+0)/383;c3 = ([120 150 230]+128)/383;patch([0 1 1 0],[0 0 1 1],c1);patch([0 1 1 1-e 1-e 0+e],[0 0 1 1-e 0+e 0+e],c2);patch([0 0 1 1-e 0+e 0+e],[0 1 1 1-e 1-e 0+e],c3);plot([0 1 1 0 0],[0 0 1 1 0]);disp('b');
  netsum : Sum  Inputs=3  SaturateOnIntegerOverflow=on  InputSameDT=on  OutDataTypeStr=Inherit: Same as first input
      mask Display: e = 0.06;c1 = [120 150 230]/255;c2 = ([120 150 230]+0)/383;c3 = ([120 150 230]+128)/383;patch([0 1 1 0],[0 0 1 1],c1);patch([0 1 1 1-e 1-e 0+e],[0 0 1 1-e 0+e 0+e],c2);patch([0 0 1 1-e 0+e 0+e],[0 1 1 1-e 1-e 0+e],c3);plot([0 1 1 0 0],[0 0 1 1 0]);disp('+');
  tansig : neural/Transfer Functions/tansig
  "a{1}" : Outport  InitialOutput=[0;0;0;0;0;0;0;0;0;0]
      mask Display: e = 0.06;c1 = [120 230 180]/255;c2 = ([120 230 180]+0)/(256+128);c3 = ([120 230 180]+128)/(256+128);patch([0 1 1 0],[0 0 1 1],c1);patch([0 1 1 1-e 1-e 0+e],[0 0 1 1-e 0+e 0+e],c2);patch([0 0 1 1-e 0+e 0+e],[0 1 1 1-e 1-e 0+e],c3);plot([0 1 1 0 0],[0 0 1 1 0]);
  wires:
  "p{1}"/1 -> Delays 1/1("p{1}")
  Delays 1/1("pd{1,1}") -> "IW{1,1}"/1("pd{1,1}")
  "IW{1,1}"/1("iz{1,1}") -> netsum/1
  "p{2}"/1 -> Delays 2/1("p{1}")
  Delays 2/1("pd{1,2}") -> "IW{1,2}"/1("pd{1,2}")
  "IW{1,2}"/1("iz{1,2}") -> netsum/2
  "b{1}"/1 -> netsum/3
  netsum/1 -> tansig/1
  tansig/1 -> "a{1}"/1

== system ball_and_plate_za_nn_2/NARX/Layer 2 ==
  "a{1} " : Inport  PortDimensions=10  SampleTime=0.001
      mask Display: e = 0.06;c1 = [120 230 180]/255;c2 = ([120 230 180]+0)/(256+128);c3 = ([120 230 180]+128)/(256+128);patch([0 1 1 0],[0 0 1 1],c1);patch([0 1 1 1-e 1-e 0+e],[0 0 1 1-e 0+e 0+e],c2);patch([0 0 1 1-e 0+e 0+e],[0 1 1 1-e 1-e 0+e],c3);plot([0 1 1 0 0],[0 0 1 1 0]);
  Delays 1 : Subsystem
      mask Display: e = 0.06;c1 = [120 150 230]/255;c2 = ([120 150 230]+0)/383;c3 = ([120 150 230]+128)/383;patch([0 1 1 0],[0 0 1 1],c1);patch([0 1 1 1-e 1-e 0+e],[0 0 1 1-e 0+e 0+e],c2);patch([0 0 1 1-e 0+e 0+e],[0 1 1 1-e 1-e 0+e],c3);plot([0 1 1 0 0],[0 0 1 1 0]);disp('0');
  "LW{2,1}" : Subsystem
      mask Display: e = 0.06;c1 = [120 150 230]/255;c2 = ([120 150 230]+0)/383;c3 = ([120 150 230]+128)/383;patch([0 1 1 0],[0 0 1 1],c1);patch([0 1 1 1-e 1-e 0+e],[0 0 1 1-e 0+e 0+e],c2);patch([0 0 1 1-e 0+e 0+e],[0 1 1 1-e 1-e 0+e],c3);plot([0 1 1 0 0],[0 0 1 1 0]);disp('W');
  "b{2}" : Constant  Value=[1.7856478998898819288143613448482938110828399658203125;-1.363202280426936141566329752095043659210205078125;1.1308291989835830282373763111536391079425811767578125;0.534348442996380956770963166491128504276275634765625;0.289070659837180998774641693671583198010921478271484375;-0.2502460788162519378374781808815896511077880859375;0.58002126559116840009977522640838287770748138427734375;0.93164667885720453543996200096444226801395416259765625;1.290621525246425260746718777227215468883514404296875;1.782219894765807222114517571753822267055511474609375]
      mask Display: e = 0.06;c1 = [120 150 230]/255;c2 = ([120 150 230]+0)/383;c3 = ([120 150 230]+128)/383;patch([0 1 1 0],[0 0 1 1],c1);patch([0 1 1 1-e 1-e 0+e],[0 0 1 1-e 0+e 0+e],c2);patch([0 0 1 1-e 0+e 0+e],[0 1 1 1-e 1-e 0+e],c3);plot([0 1 1 0 0],[0 0 1 1 0]);disp('b');
  netsum : Sum  Inputs=2  SaturateOnIntegerOverflow=on  InputSameDT=on  OutDataTypeStr=Inherit: Same as first input
      mask Display: e = 0.06;c1 = [120 150 230]/255;c2 = ([120 150 230]+0)/383;c3 = ([120 150 230]+128)/383;patch([0 1 1 0],[0 0 1 1],c1);patch([0 1 1 1-e 1-e 0+e],[0 0 1 1-e 0+e 0+e],c2);patch([0 0 1 1-e 0+e 0+e],[0 1 1 1-e 1-e 0+e],c3);plot([0 1 1 0 0],[0 0 1 1 0]);disp('+');
  tansig : neural/Transfer Functions/tansig
  "a{2}" : Outport  InitialOutput=[0;0;0;0;0;0;0;0;0;0]
      mask Display: e = 0.06;c1 = [120 230 180]/255;c2 = ([120 230 180]+0)/(256+128);c3 = ([120 230 180]+128)/(256+128);patch([0 1 1 0],[0 0 1 1],c1);patch([0 1 1 1-e 1-e 0+e],[0 0 1 1-e 0+e 0+e],c2);patch([0 0 1 1-e 0+e 0+e],[0 1 1 1-e 1-e 0+e],c3);plot([0 1 1 0 0],[0 0 1 1 0]);
  wires:
  "a{1} "/1 -> Delays 1/1("p{2}")
  Delays 1/1("pd{2,1}") -> "LW{2,1}"/1("ad{2,1}")
  "LW{2,1}"/1("lz{2,1}") -> netsum/1
  "b{2}"/1 -> netsum/2
  netsum/1 -> tansig/1
  tansig/1 -> "a{2}"/1

== system ball_and_plate_za_nn_2/NARX/Layer 3 ==
  "a{2} " : Inport  PortDimensions=10  SampleTime=0.001
      mask Display: e = 0.06;c1 = [120 230 180]/255;c2 = ([120 230 180]+0)/(256+128);c3 = ([120 230 180]+128)/(256+128);patch([0 1 1 0],[0 0 1 1],c1);patch([0 1 1 1-e 1-e 0+e],[0 0 1 1-e 0+e 0+e],c2);patch([0 0 1 1-e 0+e 0+e],[0 1 1 1-e 1-e 0+e],c3);plot([0 1 1 0 0],[0 0 1 1 0]);
  Delays 1 : Subsystem
      mask Display: e = 0.06;c1 = [120 150 230]/255;c2 = ([120 150 230]+0)/383;c3 = ([120 150 230]+128)/383;patch([0 1 1 0],[0 0 1 1],c1);patch([0 1 1 1-e 1-e 0+e],[0 0 1 1-e 0+e 0+e],c2);patch([0 0 1 1-e 0+e 0+e],[0 1 1 1-e 1-e 0+e],c3);plot([0 1 1 0 0],[0 0 1 1 0]);disp('0');
  "LW{3,2}" : Subsystem
      mask Display: e = 0.06;c1 = [120 150 230]/255;c2 = ([120 150 230]+0)/383;c3 = ([120 150 230]+128)/383;patch([0 1 1 0],[0 0 1 1],c1);patch([0 1 1 1-e 1-e 0+e],[0 0 1 1-e 0+e 0+e],c2);patch([0 0 1 1-e 0+e 0+e],[0 1 1 1-e 1-e 0+e],c3);plot([0 1 1 0 0],[0 0 1 1 0]);disp('W');
  "b{3}" : Constant  Value=[-1.7638228629634251642954723138245753943920135498046875;1.403736568653132454898013747879303991794586181640625;-1.0007086734653263260241828902508132159709930419921875;-0.456696511950927142020617566231521777808666229248046875;-0.1925083850201146640213067939839675091207027435302734375;0.30164519788435339986421013236395083367824554443359375;-0.6208600540910456100363035147893242537975311279296875;-0.9644511830031816668196142927627079188823699951171875;1.5436508687514021165299027416040189564228057861328125;1.7669298360511358492175304490956477820873260498046875]
      mask Display: e = 0.06;c1 = [120 150 230]/255;c2 = ([120 150 230]+0)/383;c3 = ([120 150 230]+128)/383;patch([0 1 1 0],[0 0 1 1],c1);patch([0 1 1 1-e 1-e 0+e],[0 0 1 1-e 0+e 0+e],c2);patch([0 0 1 1-e 0+e 0+e],[0 1 1 1-e 1-e 0+e],c3);plot([0 1 1 0 0],[0 0 1 1 0]);disp('b');
  netsum : Sum  Inputs=2  SaturateOnIntegerOverflow=on  InputSameDT=on  OutDataTypeStr=Inherit: Same as first input
      mask Display: e = 0.06;c1 = [120 150 230]/255;c2 = ([120 150 230]+0)/383;c3 = ([120 150 230]+128)/383;patch([0 1 1 0],[0 0 1 1],c1);patch([0 1 1 1-e 1-e 0+e],[0 0 1 1-e 0+e 0+e],c2);patch([0 0 1 1-e 0+e 0+e],[0 1 1 1-e 1-e 0+e],c3);plot([0 1 1 0 0],[0 0 1 1 0]);disp('+');
  tansig : neural/Transfer Functions/tansig
  "a{3}" : Outport  InitialOutput=[0;0;0;0;0;0;0;0;0;0]
      mask Display: e = 0.06;c1 = [120 230 180]/255;c2 = ([120 230 180]+0)/(256+128);c3 = ([120 230 180]+128)/(256+128);patch([0 1 1 0],[0 0 1 1],c1);patch([0 1 1 1-e 1-e 0+e],[0 0 1 1-e 0+e 0+e],c2);patch([0 0 1 1-e 0+e 0+e],[0 1 1 1-e 1-e 0+e],c3);plot([0 1 1 0 0],[0 0 1 1 0]);
  wires:
  "a{2} "/1 -> Delays 1/1("p{3}")
  Delays 1/1("pd{3,2}") -> "LW{3,2}"/1("ad{3,2}")
  "LW{3,2}"/1("lz{3,2}") -> netsum/1
  "b{3}"/1 -> netsum/2
  netsum/1 -> tansig/1
  tansig/1 -> "a{3}"/1

== system ball_and_plate_za_nn_2/NARX/Layer 4 ==
  "a{3} " : Inport  PortDimensions=10  SampleTime=0.001
      mask Display: e = 0.06;c1 = [120 230 180]/255;c2 = ([120 230 180]+0)/(256+128);c3 = ([120 230 180]+128)/(256+128);patch([0 1 1 0],[0 0 1 1],c1);patch([0 1 1 1-e 1-e 0+e],[0 0 1 1-e 0+e 0+e],c2);patch([0 0 1 1-e 0+e 0+e],[0 1 1 1-e 1-e 0+e],c3);plot([0 1 1 0 0],[0 0 1 1 0]);
  Delays 1 : Subsystem
      mask Display: e = 0.06;c1 = [120 150 230]/255;c2 = ([120 150 230]+0)/383;c3 = ([120 150 230]+128)/383;patch([0 1 1 0],[0 0 1 1],c1);patch([0 1 1 1-e 1-e 0+e],[0 0 1 1-e 0+e 0+e],c2);patch([0 0 1 1-e 0+e 0+e],[0 1 1 1-e 1-e 0+e],c3);plot([0 1 1 0 0],[0 0 1 1 0]);disp('0');
  "LW{4,3}" : Subsystem
      mask Display: e = 0.06;c1 = [120 150 230]/255;c2 = ([120 150 230]+0)/383;c3 = ([120 150 230]+128)/383;patch([0 1 1 0],[0 0 1 1],c1);patch([0 1 1 1-e 1-e 0+e],[0 0 1 1-e 0+e 0+e],c2);patch([0 0 1 1-e 0+e 0+e],[0 1 1 1-e 1-e 0+e],c3);plot([0 1 1 0 0],[0 0 1 1 0]);disp('W');
  "b{4}" : Constant  Value=[-1.73705513261448896145111575606279075145721435546875;-1.300503843080388133301994457724504172801971435546875;-0.9942067398095797425838782146456651389598846435546875;0.52099365259874674816131800980656407773494720458984375;-0.13341810709417700753220970000256784260272979736328125;0.1960689883242954234532362534082494676113128662109375;0.59537718387321236779285982265719212591648101806640625;0.96989881609432071485343840322457253932952880859375;-1.361089631891214679626500583253800868988037109375;1.729442315179101630207014750340022146701812744140625]
      mask Display: e = 0.06;c1 = [120 150 230]/255;c2 = ([120 150 230]+0)/383;c3 = ([120 150 230]+128)/383;patch([0 1 1 0],[0 0 1 1],c1);patch([0 1 1 1-e 1-e 0+e],[0 0 1 1-e 0+e 0+e],c2);patch([0 0 1 1-e 0+e 0+e],[0 1 1 1-e 1-e 0+e],c3);plot([0 1 1 0 0],[0 0 1 1 0]);disp('b');
  netsum : Sum  Inputs=2  SaturateOnIntegerOverflow=on  InputSameDT=on  OutDataTypeStr=Inherit: Same as first input
      mask Display: e = 0.06;c1 = [120 150 230]/255;c2 = ([120 150 230]+0)/383;c3 = ([120 150 230]+128)/383;patch([0 1 1 0],[0 0 1 1],c1);patch([0 1 1 1-e 1-e 0+e],[0 0 1 1-e 0+e 0+e],c2);patch([0 0 1 1-e 0+e 0+e],[0 1 1 1-e 1-e 0+e],c3);plot([0 1 1 0 0],[0 0 1 1 0]);disp('+');
  tansig : neural/Transfer Functions/tansig
  "a{4}" : Outport  InitialOutput=[0;0;0;0;0;0;0;0;0;0]
      mask Display: e = 0.06;c1 = [120 230 180]/255;c2 = ([120 230 180]+0)/(256+128);c3 = ([120 230 180]+128)/(256+128);patch([0 1 1 0],[0 0 1 1],c1);patch([0 1 1 1-e 1-e 0+e],[0 0 1 1-e 0+e 0+e],c2);patch([0 0 1 1-e 0+e 0+e],[0 1 1 1-e 1-e 0+e],c3);plot([0 1 1 0 0],[0 0 1 1 0]);
  wires:
  "a{3} "/1 -> Delays 1/1("p{4}")
  Delays 1/1("pd{4,3}") -> "LW{4,3}"/1("ad{4,3}")
  "LW{4,3}"/1("lz{4,3}") -> netsum/1
  "b{4}"/1 -> netsum/2
  netsum/1 -> tansig/1
  tansig/1 -> "a{4}"/1

== system ball_and_plate_za_nn_2/NARX/Layer 5 ==
  "a{4} " : Inport  PortDimensions=10  SampleTime=0.001
      mask Display: e = 0.06;c1 = [120 230 180]/255;c2 = ([120 230 180]+0)/(256+128);c3 = ([120 230 180]+128)/(256+128);patch([0 1 1 0],[0 0 1 1],c1);patch([0 1 1 1-e 1-e 0+e],[0 0 1 1-e 0+e 0+e],c2);patch([0 0 1 1-e 0+e 0+e],[0 1 1 1-e 1-e 0+e],c3);plot([0 1 1 0 0],[0 0 1 1 0]);
  Delays 1 : Subsystem
      mask Display: e = 0.06;c1 = [120 150 230]/255;c2 = ([120 150 230]+0)/383;c3 = ([120 150 230]+128)/383;patch([0 1 1 0],[0 0 1 1],c1);patch([0 1 1 1-e 1-e 0+e],[0 0 1 1-e 0+e 0+e],c2);patch([0 0 1 1-e 0+e 0+e],[0 1 1 1-e 1-e 0+e],c3);plot([0 1 1 0 0],[0 0 1 1 0]);disp('0');
  "LW{5,4}" : Subsystem
      mask Display: e = 0.06;c1 = [120 150 230]/255;c2 = ([120 150 230]+0)/383;c3 = ([120 150 230]+128)/383;patch([0 1 1 0],[0 0 1 1],c1);patch([0 1 1 1-e 1-e 0+e],[0 0 1 1-e 0+e 0+e],c2);patch([0 0 1 1-e 0+e 0+e],[0 1 1 1-e 1-e 0+e],c3);plot([0 1 1 0 0],[0 0 1 1 0]);disp('W');
  "b{5}" : Constant  Value=0.033345244642292527770255361474482924677431583404541015625
      mask Display: e = 0.06;c1 = [120 150 230]/255;c2 = ([120 150 230]+0)/383;c3 = ([120 150 230]+128)/383;patch([0 1 1 0],[0 0 1 1],c1);patch([0 1 1 1-e 1-e 0+e],[0 0 1 1-e 0+e 0+e],c2);patch([0 0 1 1-e 0+e 0+e],[0 1 1 1-e 1-e 0+e],c3);plot([0 1 1 0 0],[0 0 1 1 0]);disp('b');
  netsum : Sum  Inputs=2  SaturateOnIntegerOverflow=on  InputSameDT=on  OutDataTypeStr=Inherit: Same as first input
      mask Display: e = 0.06;c1 = [120 150 230]/255;c2 = ([120 150 230]+0)/383;c3 = ([120 150 230]+128)/383;patch([0 1 1 0],[0 0 1 1],c1);patch([0 1 1 1-e 1-e 0+e],[0 0 1 1-e 0+e 0+e],c2);patch([0 0 1 1-e 0+e 0+e],[0 1 1 1-e 1-e 0+e],c3);plot([0 1 1 0 0],[0 0 1 1 0]);disp('+');
  purelin : neural/Transfer Functions/purelin
  "a{5}" : Outport  InitialOutput=0
      mask Display: e = 0.06;c1 = [120 230 180]/255;c2 = ([120 230 180]+0)/(256+128);c3 = ([120 230 180]+128)/(256+128);patch([0 1 1 0],[0 0 1 1],c1);patch([0 1 1 1-e 1-e 0+e],[0 0 1 1-e 0+e 0+e],c2);patch([0 0 1 1-e 0+e 0+e],[0 1 1 1-e 1-e 0+e],c3);plot([0 1 1 0 0],[0 0 1 1 0]);
  wires:
  "a{4} "/1 -> Delays 1/1("p{5}")
  Delays 1/1("pd{5,4}") -> "LW{5,4}"/1("ad{5,4}")
  "LW{5,4}"/1("lz{5,4}") -> netsum/1
  "b{5}"/1 -> netsum/2
  netsum/1 -> purelin/1
  purelin/1 -> "a{5}"/1

== system ball_and_plate_za_nn_2/NARX/Process Input 1 ==
  x : Inport  PortDimensions=1  SampleTime=0.001
      mask Display: e = 0.06;c1 = [120 230 180]/255;c2 = ([120 230 180]+0)/(256+128);c3 = ([120 230 180]+128)/(256+128);patch([0 1 1 0],[0 0 1 1],c1);patch([0 1 1 1-e 1-e 0+e],[0 0 1 1-e 0+e 0+e],c2);patch([0 0 1 1-e 0+e 0+e],[0 1 1 1-e 1-e 0+e],c3);plot([0 1 1 0 0],[0 0 1 1 0]);
  mapminmax : neural/Processing Functions/mapminmax  xmin=-4.93752318466582895695182742202  xmax=4.56655998973498622461875129375  ymin=-1  ymax=1
  p : Outport  PortDimensions=1  SampleTime=0.001
      mask Display: e = 0.06;c1 = [120 230 180]/255;c2 = ([120 230 180]+0)/(256+128);c3 = ([120 230 180]+128)/(256+128);patch([0 1 1 0],[0 0 1 1],c1);patch([0 1 1 1-e 1-e 0+e],[0 0 1 1-e 0+e 0+e],c2);patch([0 0 1 1-e 0+e 0+e],[0 1 1 1-e 1-e 0+e],c3);plot([0 1 1 0 0],[0 0 1 1 0]);
  wires:
  x/1 -> mapminmax/1
  mapminmax/1 -> p/1

== system ball_and_plate_za_nn_2/NARX/Process Input 2 ==
  x : Inport  PortDimensions=1  SampleTime=0.001
      mask Display: e = 0.06;c1 = [120 230 180]/255;c2 = ([120 230 180]+0)/(256+128);c3 = ([120 230 180]+128)/(256+128);patch([0 1 1 0],[0 0 1 1],c1);patch([0 1 1 1-e 1-e 0+e],[0 0 1 1-e 0+e 0+e],c2);patch([0 0 1 1-e 0+e 0+e],[0 1 1 1-e 1-e 0+e],c3);plot([0 1 1 0 0],[0 0 1 1 0]);
  mapminmax : neural/Processing Functions/mapminmax  xmin=-0.0186760527491309710756972606305  xmax=0.477601634373471639616326456235  ymin=-1  ymax=1
  p : Outport  PortDimensions=1  SampleTime=0.001
      mask Display: e = 0.06;c1 = [120 230 180]/255;c2 = ([120 230 180]+0)/(256+128);c3 = ([120 230 180]+128)/(256+128);patch([0 1 1 0],[0 0 1 1],c1);patch([0 1 1 1-e 1-e 0+e],[0 0 1 1-e 0+e 0+e],c2);patch([0 0 1 1-e 0+e 0+e],[0 1 1 1-e 1-e 0+e],c3);plot([0 1 1 0 0],[0 0 1 1 0]);
  wires:
  x/1 -> mapminmax/1
  mapminmax/1 -> p/1

== system ball_and_plate_za_nn_2/NARX/Process Output 1 ==
  a : Inport  PortDimensions=1  SampleTime=0.001
      mask Display: e = 0.06;c1 = [120 230 180]/255;c2 = ([120 230 180]+0)/(256+128);c3 = ([120 230 180]+128)/(256+128);patch([0 1 1 0],[0 0 1 1],c1);patch([0 1 1 1-e 1-e 0+e],[0 0 1 1-e 0+e 0+e],c2);patch([0 0 1 1-e 0+e 0+e],[0 1 1 1-e 1-e 0+e],c3);plot([0 1 1 0 0],[0 0 1 1 0]);
  mapminmax_reverse : neural/Processing Functions/mapminmax_reverse  xmin=-0.0186760527491309710756972606305  xmax=0.477601634373471639616326456235  ymin=-1  ymax=1
  y : Outport  PortDimensions=1  SampleTime=0.001
      mask Display: e = 0.06;c1 = [120 230 180]/255;c2 = ([120 230 180]+0)/(256+128);c3 = ([120 230 180]+128)/(256+128);patch([0 1 1 0],[0 0 1 1],c1);patch([0 1 1 1-e 1-e 0+e],[0 0 1 1-e 0+e 0+e],c2);patch([0 0 1 1-e 0+e 0+e],[0 1 1 1-e 1-e 0+e],c3);plot([0 1 1 0 0],[0 0 1 1 0]);
  wires:
  a/1 -> mapminmax_reverse/1
  mapminmax_reverse/1 -> y/1
